simulink model "L_21_05_12_Esercizio_progetto_di_un_controllore_schema"  (R2021a)
settings: Solver=VariableStepAuto  StartTime=0.0  StopTime=10.0  RelTol=1e-3
values from neighbouring files (symbols this model uses):
  Kr = 1    [L_11_05_21_reti_anticipatrici.m]    (also in L_11_05_21_reti_anticipatrici_2.m; L_12_05_21_Esercizio_progetto_di_un_controllore.m; L_12_05_21_effetti_sul_comando.m; L_12_05_21_reti_integro-derivative.m)
libraries: cstblocks x3, simulink x1
settings Model: Creator=armandofornasier  LastModifiedBy=armandofornasier

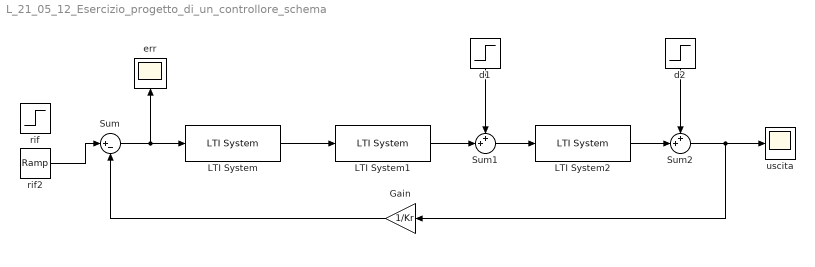
== system L_21_05_12_Esercizio_progetto_di_un_controllore_schema ==
  Gain : Gain  Gain=1/Kr
  LTI System : cstblocks/LTI System  sys=C  IC=[]
  LTI System1 : cstblocks/LTI System  sys=F1  IC=[]
  LTI System2 : cstblocks/LTI System  sys=F2  IC=[]
  Sum : Sum  Inputs=|+-
  Sum1 : Sum  Inputs=++|
  Sum2 : Sum  Inputs=++|
  d1 : Step  Time=0  After=0.5  SampleTime=0
  d2 : Step  Time=0  After=0.2  SampleTime=0
  err : Scope
  rif : Step  SampleTime=0
  rif2 : simulink/Sources/Ramp  slope=0  start=0  InitialOutput=0
  uscita : Scope
  wires:
  Sum/1 -> err/1, LTI System/1
  LTI System/1 -> LTI System1/1
  Sum1/1 -> LTI System2/1
  LTI System1/1 -> Sum1/2
  LTI System2/1 -> Sum2/2
  Sum2/1 -> Gain/1, uscita/1
  Gain/1 -> Sum/2
  rif2/1 -> Sum/1
  d2/1 -> Sum2/1
  d1/1 -> Sum1/1
